simulink model "MalhaAberta"  (Simulink 7.7)
settings: Solver=ode45  StartTime=0.0  StopTime=4000  RelTol=1e-3
values from neighbouring files (symbols this model uses):
  QT =     [FaseMinima.mat]    (also in FaseNaoMinima.mat; FaseNaoMinimaMudandoApenasGama.mat; settup.m = dynamics())
settings Model: Creator=Arthur  LastModifiedBy=Arthur

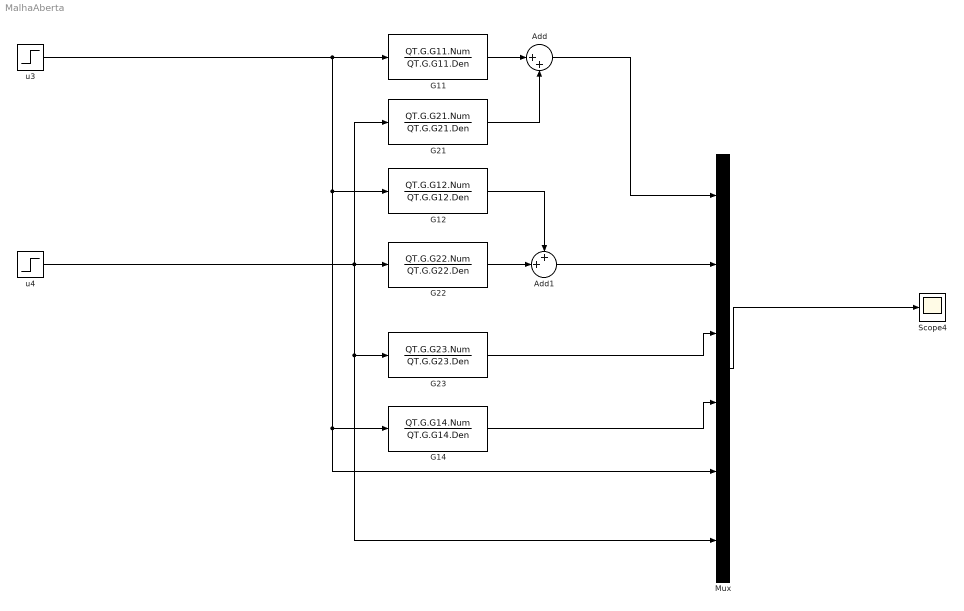
== system MalhaAberta ==
  Add : Sum  Inputs=|++
  Add1 : Sum  Inputs=++|
  G11 : TransferFcn  Numerator=QT.G.G11.Num  Denominator=QT.G.G11.Den
  G12 : TransferFcn  Numerator=QT.G.G12.Num  Denominator=QT.G.G12.Den
  G14 : TransferFcn  Numerator=QT.G.G14.Num  Denominator=QT.G.G14.Den
  G21 : TransferFcn  Numerator=QT.G.G21.Num  Denominator=QT.G.G21.Den
  G22 : TransferFcn  Numerator=QT.G.G22.Num  Denominator=QT.G.G22.Den
  G23 : TransferFcn  Numerator=QT.G.G23.Num  Denominator=QT.G.G23.Den
  Mux : Mux  Inputs=6
  Scope4 : Scope
      settings: TimeRange=10  SaveName=SimuladoNM
  u3 : Step  Time=100  After=0.15  SampleTime=0
  u4 : Step  Time=1400  After=0.15  SampleTime=0
  wires:
  G11/1 -> Add/1
  G21/1 -> Add/2
  G22/1 -> Add1/2
  G12/1 -> Add1/1
  Add/1 -> Mux/1
  u3/1 -> G11/1, G12/1, G14/1, Mux/5
  u4/1 -> G22/1, G21/1, G23/1, Mux/6
  Add1/1 -> Mux/2
  Mux/1 -> Scope4/1
  G23/1 -> Mux/3
  G14/1 -> Mux/4
